simulink model "turbofanmatch"  (R2018a)
settings: Solver=VariableStepAuto  StartTime=0.0  StopTime=0.0  RelTol=1e-3
libraries: motorlib x12
settings Model: Creator=mairon  LastModifiedBy=mairon

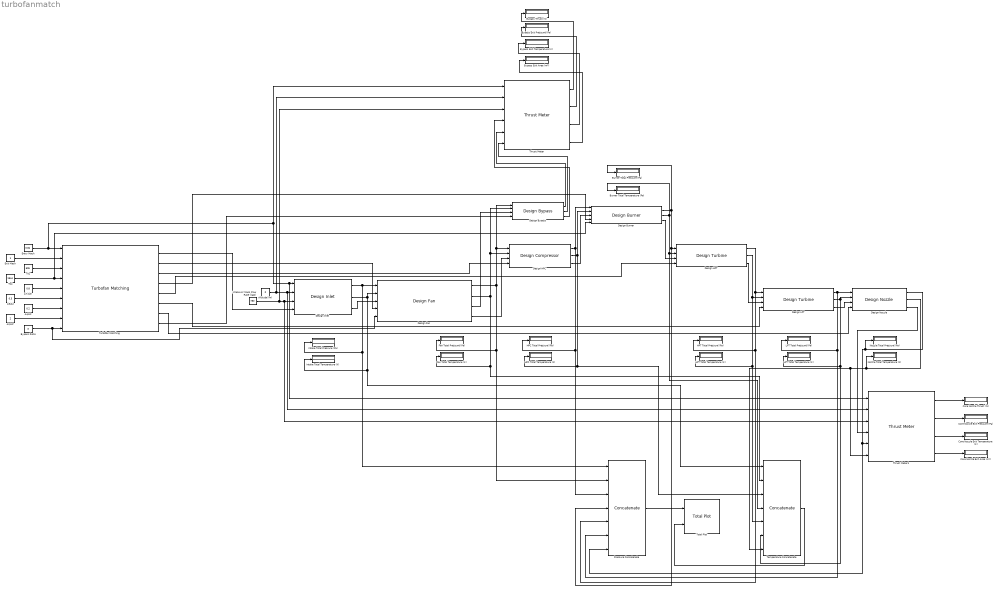
== system turbofanmatch ==
  A2/A2' : Constant  Value=2
  A4/A2 : Constant  Value=0.2
  A5/A2 : Constant  Value=0.3
  A7'/A3' : Constant  Value=0.8
  Altitude (m) : Constant  Value=0
  Burner Total Pressure (Pa) : Display
  Burner Total Temperature (Pa) : Display
  Bypass Exit Area (m²) : Display
  Bypass Exit Pressure (Pa) : Display
  Bypass Exit Temperature (K) : Display
  Bypass Ratio : Constant  Value=3
  Bypass Thrust (N) : Display
  Core Nozzle Exit Area (m²) : Display
  Core Nozzle Exit Pressure (Pa) : Display
  Core Nozzle Exit Temperature (K) : Display
  Core Nozzle Thrust (N) : Display
  Design Burner : motorlib/Design Burner
      settings: SourceProductName=Aeronautic Motor
  Design Bypass : motorlib/Design Bypass
      settings: SourceProductName=Aeronautic Motor
  Design Fan : motorlib/Design Fan
      settings: SourceProductName=Aeronautic Motor
  Design HPC : motorlib/Design Compressor
      settings: SourceProductName=Aeronautic Motor
  Design HPT : motorlib/Design Turbine
      settings: SourceProductName=Aeronautic Motor
  Design Inlet : motorlib/Design Inlet
      settings: SourceProductName=Aeronautic Motor
  Design LPT : motorlib/Design Turbine
      settings: SourceProductName=Aeronautic Motor
  Design Nozzle : motorlib/Design Nozzle
      settings: SourceProductName=Aeronautic Motor
  Entry Mach : Constant  Value=0.84
  Exit Mach : Constant
  Fan Total Pressure (Pa) : Display
  Fan Total Temperature (K) : Display
  HPC Total Pressure (Pa) : Display
  HPC Total Temperature (K) : Display
  HPT Total Pressure (Pa) : Display
  HPT Total Temperature (K) : Display
  Intake Air Mass Flow Rate (kg/s) : Constant  Value=780
  Intake Total Pressure (Pa) : Display
  Intake Total Temperature (K) : Display
  LPT Total Pressure (Pa) : Display
  LPT Total Temperature (K) : Display
  Nozzle Total Pressure (Pa) : Display
  Nozzle Total Temperature (K) : Display
  Pressure Concatenate : Concatenate  NumInputs=7
  Temperature Concatenate : Concatenate  NumInputs=7
  Thrust Meter : motorlib/Thrust Meter
      settings: SourceProductName=Aeronautic Motor
  Thrust Meter1 : motorlib/Thrust Meter
      settings: SourceProductName=Aeronautic Motor
  To2 : Constant  Value=605
  To4 : Constant  Value=1944
  Total Plot : motorlib/Total Plot
      settings: SourceProductName=Aeronautic Motor
  Turbofan Matching : motorlib/Turbofan Matching
      settings: SourceProductName=Aeronautic Motor
  wires:
  Design Inlet/1 -> Pressure Concatenate/1, Intake Total Pressure (Pa)/1, Design Fan/1
  Design Inlet/2 -> Design Fan/2, Temperature Concatenate/1, Intake Total Temperature (K)/1
  Design HPC/1 -> Design Burner/1, HPC Total Pressure (Pa)/1, Pressure Concatenate/3
  Design HPC/2 -> Design Burner/2, Temperature Concatenate/3, HPC Total Temperature (K)/1
  Design Burner/1 -> Pressure Concatenate/4, Design HPT/1, Burner Total Pressure (Pa)/1
  Design Burner/2 -> Temperature Concatenate/4, Design HPT/2, Burner Total Temperature (Pa)/1
  Design Burner/3 -> Design HPT/3
  Design HPT/1 -> Design LPT/1, Pressure Concatenate/5, HPT Total Pressure (Pa)/1
  Design HPT/2 -> Design LPT/2, Temperature Concatenate/5, HPT Total Temperature (K)/1
  Design HPT/3 -> Design LPT/3
  Design LPT/1 -> Design Nozzle/1, Pressure Concatenate/6, LPT Total Pressure (Pa)/1
  Design LPT/2 -> Design Nozzle/2, Temperature Concatenate/6, LPT Total Temperature (K)/1
  Design LPT/3 -> Design Nozzle/3
  Altitude (m)/1 -> Thrust Meter/2, Thrust Meter1/2, Design Inlet/2
  Entry Mach/1 -> Thrust Meter1/1, Design Inlet/1, Thrust Meter/1, Turbofan Matching/1
  Design Fan/1 -> Pressure Concatenate/2, Fan Total Pressure (Pa)/1, Design Bypass/1, Design HPC/1
  Design Nozzle/1 -> Pressure Concatenate/7, Thrust Meter1/5, Nozzle Total Pressure (Pa)/1
  Design Nozzle/2 -> Temperature Concatenate/7, Thrust Meter1/6, Nozzle Total Temperature (K)/1
  Design Inlet/3 -> Design Fan/3
  Design Fan/2 -> Temperature Concatenate/2, Fan Total Temperature (K)/1, Design Bypass/2, Design HPC/2
  Design Bypass/1 -> Thrust Meter/5
  Design Bypass/2 -> Thrust Meter/6
  Design Bypass/3 -> Thrust Meter/4
  Thrust Meter/1 -> Bypass Thrust (N)/1
  Thrust Meter/2 -> Bypass Exit Pressure (Pa)/1
  Thrust Meter/3 -> Bypass Exit Temperature (K)/1
  Thrust Meter/4 -> Bypass Exit Area (m²)/1
  Design Nozzle/3 -> Thrust Meter1/4
  Thrust Meter1/1 -> Core Nozzle Thrust (N)/1
  Thrust Meter1/2 -> Core Nozzle Exit Pressure (Pa)/1
  Thrust Meter1/3 -> Core Nozzle Exit Temperature (K)/1
  Thrust Meter1/4 -> Core Nozzle Exit Area (m²)/1
  Pressure Concatenate/1 -> Total Plot/1
  Temperature Concatenate/1 -> Total Plot/2
  Exit Mach/1 -> Turbofan Matching/2
  To2/1 -> Turbofan Matching/3
  To4/1 -> Design Burner/5, Turbofan Matching/4
  A7'/A3'/1 -> Turbofan Matching/5
  A5/A2/1 -> Turbofan Matching/6
  A4/A2/1 -> Turbofan Matching/7
  A2/A2'/1 -> Turbofan Matching/8
  Bypass Ratio/1 -> Design Fan/5, Turbofan Matching/9
  Intake Air Mass Flow Rate (kg/s)/1 -> Thrust Meter/3, Thrust Meter1/3, Design Inlet/3
  Turbofan Matching/1 -> Design Inlet/4
  Design Fan/4 -> Design HPC/3
  Design Fan/3 -> Design Bypass/3
  Turbofan Matching/2 -> Design Fan/4
  Design HPC/3 -> Design Burner/3
  Turbofan Matching/3 -> Design HPC/4
  Turbofan Matching/8 -> Design Bypass/4
  Turbofan Matching/4 -> Design Burner/4
  Turbofan Matching/5 -> Design HPT/4
  Turbofan Matching/6 -> Design LPT/4
  Turbofan Matching/7 -> Design Nozzle/4
